simulink model "Winda_2015b"  (R2016a)
settings: Solver=FixedStepDiscrete  StartTime=0.0  StopTime=40  FixedStep=0.05  MaxStep=0.1  MinStep=0.01  RelTol=1e-3
undefined symbols (not defined in the file or in its folder): sigbuilder_block
libraries: simulink x12
settings Model: Creator=dmar  LastModifiedBy=Piotr
settings DataIOCC: LimitDataPoints=on  SaveFormat=Array  SignalLoggingSaveFormat=ModelDataLogs
settings OptimizationCC: ExpressionDepthLimit=2147483647
settings DebuggingCC: UnderspecifiedInitializationDetection=Classic  MergeDetectMultiDrivingBlocksExec=none  SolverPrmCheckMsg=warning  ParameterPrecisionLossMsg=none  FcnCallInpInsideContextMsg=UseLocalSettings  AllowSymbolicDim=off  StateNameClashWarn=warning
settings HardwareCC: ProdBitPerPointer=32  ProdLargestAtomicFloat=None  ProdIntDivRoundTo=Undefined  ProdEndianess=Unspecified  ProdWordSize=32  ProdHWDeviceType=32-bit Generic
settings ModelReferenceCC: PropagateSignalLabelsOutOfModel=off
settings SFSimCC: SimParseCustomCode=off
settings GRTTargetCC: CombineOutputUpdateFcns=off  GRTInterface=on
settings ConfigComp: CovModelRefEnable=Off

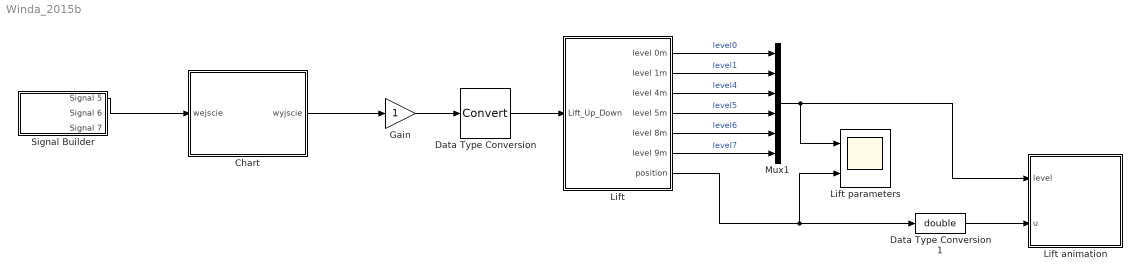
== system Winda_2015b ==
  Chart : Stateflow chart  TreatAsAtomicUnit=on
  Data Type Conversion : DataTypeConversion
  Data Type Conversion1 : DataTypeConversion  OutDataTypeStr=double
  Gain : Gain
  Lift : Subsystem
  Lift animation : MATLAB Function  TreatAsAtomicUnit=on  SystemSampleTime=0.05
  Lift parameters : Scope  NumInputPorts=2
  Mux1 : Mux  Inputs=6
  Signal Builder : Subsystem  Tag=STV Subsys  LoadFcn=sigbuilder_block('load',[153 78 550.5 394.5 ]);  StartFcn=sigbuilder_block('start');  StopFcn=sigbuilder_block('stop');  ClipboardFcn=sigbuilder_block('clipboard');  mask(Sigbuilder block){}
      mask help: Simulink:masks:SigbuilderBlock_MD
      mask init:
      | if ~strcmp(get_param(bdroot(gcbh),'SimulationStatus'),'stopped') tuvar = sigbuilder_block('maskInit'); end
      settings: CopyFcn=sigbuilder_block('copy');  DeleteFcn=sigbuilder_block('delete');  ModelCloseFcn=sigbuilder_block('modelClose');  PreSaveFcn=sigbuilder_block('preSave');  PauseFcn=sigbuilder_block('pause');  ContinueFcn=sigbuilder_block('continue');  NameChangeFcn=sigbuilder_block('namechange');  OpenFcn=sigbuilder_block('open',[153 78 550.5 394.5 ]);  CloseFcn=sigbuilder_block('close');
      mask Display: plot(0, 0, 100, 100,[2, 2, 32, 32, 2], [68, 8, 8, 68, 68],[32, 2], [38, 38], [32, 19, 2],[53, 60, 44], [32, 17, 17, 2],[16, 16, 31, 31]);txt = getActiveGroup(gcbh);text(2, 100, txt,'verticalAlignment', 'top');
  wires:
  Lift/7(position) -> Lift parameters/2, Data Type Conversion1/1
  Gain/1 -> Data Type Conversion/1
  Mux1/1 -> Lift parameters/1, Lift animation/1(level)
  Lift/1(level 0m) -> Mux1/1  "level0"
  Lift/2(level 1m) -> Mux1/2  "level1"
  Lift/3(level 4m) -> Mux1/3  "level4"
  Lift/4(level 5m) -> Mux1/4  "level5"
  Lift/5(level 8m) -> Mux1/5  "level6"
  Lift/6(level 9m) -> Mux1/6  "level7"
  Data Type Conversion/1 -> Lift/1(Lift_Up_Down)
  Data Type Conversion1/1 -> Lift animation/2(u)
  Chart/1(wyjscie) -> Gain/1
  Signal Builder/1(Signal 5) -> Chart/1(wejscie)

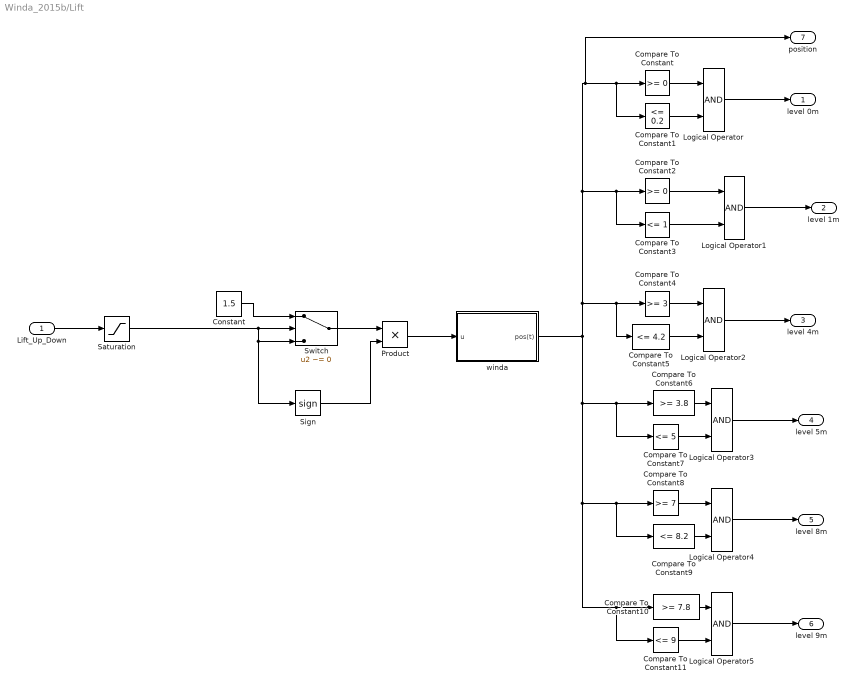
== system Winda_2015b/Lift ==
  Lift_Up_Down : Inport
  Compare To Constant : simulink/Logic and Bit Operations/Compare To Constant  relop=>=  const=0  OutDataTypeStr=boolean
  Compare To Constant1 : simulink/Logic and Bit Operations/Compare To Constant  relop=<=  const=0.2  OutDataTypeStr=boolean
  Compare To Constant10 : simulink/Logic and Bit Operations/Compare To Constant  relop=>=  const=7.8  OutDataTypeStr=boolean
  Compare To Constant11 : simulink/Logic and Bit Operations/Compare To Constant  relop=<=  const=9  OutDataTypeStr=boolean
  Compare To Constant2 : simulink/Logic and Bit Operations/Compare To Constant  relop=>=  const=0  OutDataTypeStr=boolean
  Compare To Constant3 : simulink/Logic and Bit Operations/Compare To Constant  relop=<=  const=1  OutDataTypeStr=boolean
  Compare To Constant4 : simulink/Logic and Bit Operations/Compare To Constant  relop=>=  const=3  OutDataTypeStr=boolean
  Compare To Constant5 : simulink/Logic and Bit Operations/Compare To Constant  relop=<=  const=4.2  OutDataTypeStr=boolean
  Compare To Constant6 : simulink/Logic and Bit Operations/Compare To Constant  relop=>=  const=3.8  OutDataTypeStr=boolean
  Compare To Constant7 : simulink/Logic and Bit Operations/Compare To Constant  relop=<=  const=5  OutDataTypeStr=boolean
  Compare To Constant8 : simulink/Logic and Bit Operations/Compare To Constant  relop=>=  const=7  OutDataTypeStr=boolean
  Compare To Constant9 : simulink/Logic and Bit Operations/Compare To Constant  relop=<=  const=8.2  OutDataTypeStr=boolean
  Constant : Constant  Value=1.5
  Logical Operator{,1..5} (6 alike) : Logic  AllPortsSameDT=off  OutDataTypeStr=boolean
  Product : Product  OutDataTypeStr=Inherit: Inherit via back propagation  RndMeth=Zero
  Saturation : Saturate  UpperLimit=1  LowerLimit=-1
  Sign : Signum
  Switch : Switch  Criteria=u2 ~= 0  OutDataTypeStr=Inherit: Inherit via back propagation
  winda : Subsystem
  level 0m : Outport
  level 1m : Outport  Port=2
  level 4m : Outport  Port=3
  level 5m : Outport  Port=4
  level 8m : Outport  Port=5
  level 9m : Outport  Port=6
  position : Outport  Port=7
  wires:
  Constant/1 -> Switch/1
  Lift_Up_Down/1 -> Saturation/1
  Switch/1 -> Product/1
  Product/1 -> winda/1(u)
  Sign/1 -> Product/2
  Logical Operator/1 -> level 0m/1
  Compare To Constant/1 -> Logical Operator/1
  Compare To Constant1/1 -> Logical Operator/2
  Logical Operator1/1 -> level 1m/1
  Compare To Constant2/1 -> Logical Operator1/1
  Compare To Constant3/1 -> Logical Operator1/2
  Logical Operator2/1 -> level 4m/1
  Compare To Constant4/1 -> Logical Operator2/1
  Compare To Constant5/1 -> Logical Operator2/2
  Logical Operator3/1 -> level 5m/1
  Compare To Constant6/1 -> Logical Operator3/1
  Compare To Constant7/1 -> Logical Operator3/2
  Logical Operator4/1 -> level 8m/1
  Compare To Constant8/1 -> Logical Operator4/1
  Compare To Constant9/1 -> Logical Operator4/2
  Logical Operator5/1 -> level 9m/1
  winda/1(pos(t)) -> position/1, Compare To Constant1/1, Compare To Constant/1, Compare To Constant2/1, Compare To Constant3/1, Compare To Constant5/1, Compare To Constant4/1, Compare To Constant10/1, Compare To Constant11/1, Compare To Constant9/1, Compare To Constant8/1, Compare To Constant6/1, Compare To Constant7/1
  Compare To Constant10/1 -> Logical Operator5/1
  Compare To Constant11/1 -> Logical Operator5/2
  Saturation/1 -> Sign/1, Switch/3, Switch/2

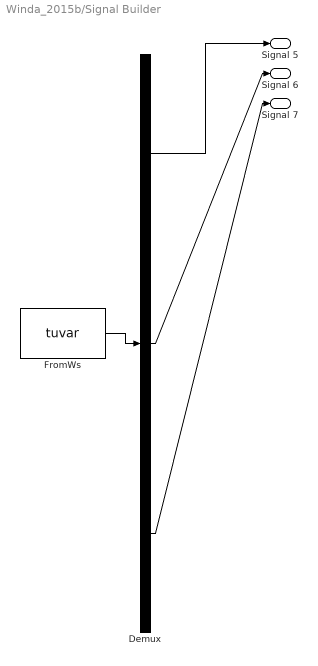
== system Winda_2015b/Signal Builder ==
  Demux : Demux  Tag=STV Demux  Outputs=3
  FromWs : FromWorkspace  Tag=STV FromWs  VariableName=tuvar  SampleTime=0
      SigBuilderData=|
      | common.afterFinalStr = 'Extrapolate'
      | common.sampleTime = 0
      | dataSet.timeRange = [0 40]
      | dataSet.name = 'Wew'
      | sbobj.Groups.Name = 'Wew'
      | sbobj.Groups.Signals(1).Name = 'Signal 5'
      | sbobj.Groups.Signals(1).XData = [0 10 10 20.1 20.1 30 40]
      | sbobj.Groups.Signals(1).YData = [0 0 1 1 0 0 0]
      | sbobj.Groups.Signals(2).Name = 'Signal 6'
      | sbobj.Groups.Signals(2).XData = [0 16 16 24 24 40]
      | sbobj.Groups.Signals(2).YData = [0 0 1 1 0 0]
      | sbobj.Groups.Signals(3).Name = 'Signal 7'
      | sbobj.Groups.Signals(3).XData = [0 16 16 24 24 40]
      | sbobj.Groups.Signals(3).YData = [0 0 1 1 0 0]
      | sbobj.Groups.TimeRange = [0 40]
  Signal 5 : Outport  Tag=STV Outport
  Signal 6 : Outport  Tag=STV Outport  Port=2
  Signal 7 : Outport  Tag=STV Outport  Port=3
  wires:
  Demux/1 -> Signal 5/1
  FromWs/1 -> Demux/1
  Demux/2 -> Signal 6/1
  Demux/3 -> Signal 7/1

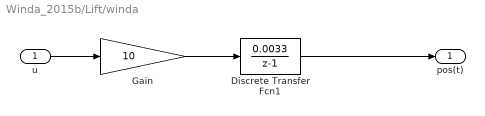
== system Winda_2015b/Lift/winda ==
  u : Inport
  Discrete Transfer Fcn1 : DiscreteTransferFcn  Numerator=[0.0033]  Denominator=[1 -1]  SampleTime=0.05  StateDataTypeStr=fixdt(1,26,12)  NumCoefDataTypeStr=fixdt(1,26,12)  DenCoefDataTypeStr=fixdt(1,26,12)  NumProductDataTypeStr=fixdt(1,26,12)  DenProductDataTypeStr=fixdt(1,26,12)  NumAccumDataTypeStr=fixdt(1,26,12)  DenAccumDataTypeStr=fixdt(1,26,12)  OutDataTypeStr=fixdt(1,26,12)
  Gain : Gain  Gain=10  ParamDataTypeStr=fixdt(1,15,2)  OutDataTypeStr=Inherit: Same as input
  pos(t) : Outport
  wires:
  u/1 -> Gain/1
  Gain/1 -> Discrete Transfer Fcn1/1
  Discrete Transfer Fcn1/1 -> pos(t)/1

== matlab function Winda_2015b/Lift animation ==
  data: level input; u input
function plot_Lift3( level,u)
%#codegen




persistent fig3;
persistent NOWE1;
persistent L_pos;


if isempty(L_pos),

    if isempty(fig3), 
    fig3 = figure(3);
    else
    close(fig3);
    fig3 = figure(3);
    end
     %NOWE1 = [0 0.1 0.1 0 0; 0.25 .25 0 0 .25]*10;
    NOWE1 = [.1 0 0 .1 .1 .09 .09 .1; 0 0 0.25 0.25 0 0 0.12 .12]*10;
    
    axis([-4 4 -1 15]);
    grid('off');
    %xlabel('X position [m]');
    ylabel('Lift position [m]');
    hold('on');
    line([-0.05 -0.05],[0 12],'LineWidth',2,'Color','k')
    line([1.05 1.05],[0 12],'LineWidth',2,'Color','k')
    line([-4 4],[-0.05 -0.05],'LineWidth',2,'Color','k')
    
    line([-1 -0.05],[4 4],'LineWidth',2,'Color','k')
    line([1.05 2],[4 4],'LineWidth',2,'Color','k')
    
    line([-1 -0.05],[8 8],'LineWidth',2,'Color','k')
    line([1.05 2],[8 8],'LineWidth',2,'Color','k')
    
    line([-1 -0.05],[12 12],'LineWidth',2,'Color','k')
    line([1.05 2],[12 12],'LineWidth',2,'Color','k')
    
 % czarna lampka na wysokosci 0
 line([1.05 1.2],[0.2 0.2],'LineWidth',4,'Color','k')

 % czarna lampka na wysokosci 1
 line([1.05 1.2],[1 1],'LineWidth',4,'Color','k')
    
 % czarna lampka na wysokosci 4
 line([1.05 1.2],[4 4],'LineWidth',4,'Color','k')

 % czarna lampka na wysokosci 5
 line([1.05 1.2],[5 5],'LineWidth',4,'Color','k')
    
  % czarna lampka na wysokosci 8
 line([1.05 1.2],[8 8],'LineWidth',4,'Color','k')
 % czarna lampka na wysokosci 9
 line([1.05 1.2],[9 9],'LineWidth',4,'Color','k')
   
%plot(NOWE1(1,:),NOWE1(2,:)+prev1,'w');
L_pos=plot(NOWE1(1,:),NOWE1(2,:)+u,'b');
    
    
    
else
    if(ishghandle(L_pos)),
       
        set(L_pos,'yData',NOWE1(2,:)+u);


if level(1)==1    
 % czarna lampka na wysokosci 0
 line([1.05 1.2],[0.2 0.2],'LineWidth',4,'Color','r');
else
 line([1.05 1.2],[0.2 0.2],'LineWidth',4,'Color','k');
end

if level(2)==1    
 % czarna lampka na wysokosci 1
 line([1.05 1.2],[1 1],'LineWidth',4,'Color','r');
else
 line([1.05 1.2],[1 1],'LineWidth',4,'Color','k');
end

if level(3)==1    
 % czarna lampka na wysokosci 4
 line([1.05 1.2],[4 4],'LineWidth',4,'Color','r');
else
 line([1.05 1.2],[4 4],'LineWidth',4,'Color','k');
end

if level(4)==1    
 % czarna lampka na wysokosci 5
 line([1.05 1.2],[5 5],'LineWidth',4,'Color','r');
else
 line([1.05 1.2],[5 5],'LineWidth',4,'Color','k');
end

if level(5)==1    
 % czarna lampka na wysokosci 8
 line([1.05 1.2],[8 8],'LineWidth',4,'Color','r');
else
 line([1.05 1.2],[8 8],'LineWidth',4,'Color','k');
end

if level(6)==1    
 % czarna lampka na wysokosci 9
 line([1.05 1.2],[9 9],'LineWidth',4,'Color','r');
else
 line([1.05 1.2],[9 9],'LineWidth',4,'Color','k');
end



     
        
        
        
    end,
end

== stateflow chart Winda_2015b/Chart ==
  state level_3
  state level_2_3
  state level_2
  state level_1_2
  state level_1
  level_2_3 -> level_3 [order 1]
  level_3 -> level_2_3
  level_2_3 -> level_2 [order 2]
  level_2 -> level_2_3 [order 1]
  level_1_2 -> level_2 [order 1]
  level_2 -> level_1_2 [order 2]
  level_1_2 -> level_1 [order 2]
  (default) -> level_1
  level_1 -> level_1_2
  data: wejscie input; wyjscie output
